simulink model "Trí"  (R2019a)
settings: Solver=FixedStepAuto  StartTime=0.0  StopTime=15  FixedStep=0.01  RelTol=1e-3
model workspace (MATLAB code in the model file):
  | Assem_DataFile.m
undefined symbols (not defined in the file): smiData, X, Y, Z
libraries: sm_lib x272, simulink x8, nesl_utility x8
(part 1 of 6)
settings Model: EnablePacing=on  Creator=DELL  LastModifiedBy=Minh Trí

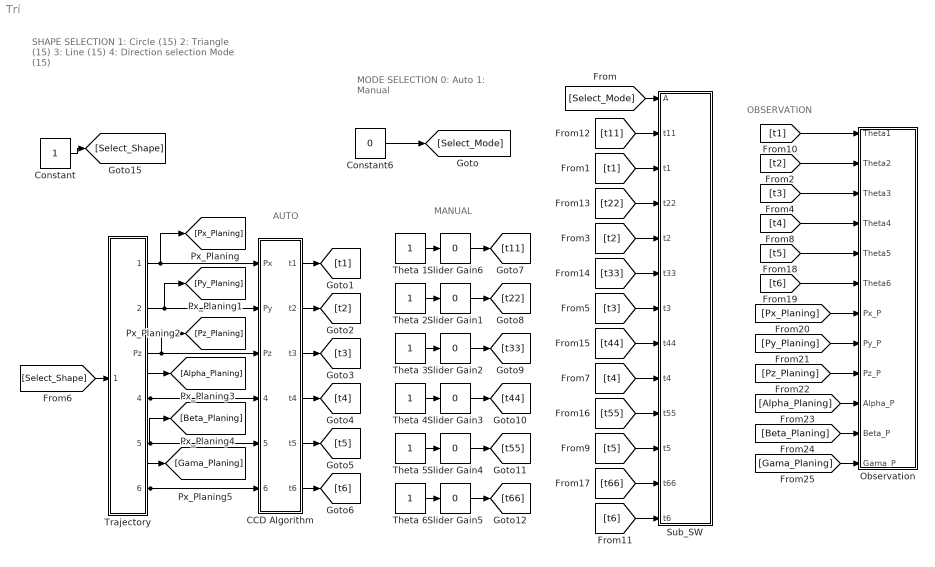
== system Trí ==
  note: MANUAL
  note: AUTO
  note: MODE SELECTION
      | 0: Auto
      | 1: Manual
  note: SHAPE SELECTION
      | 1: Circle (15)
      | 2: Triangle (15)
      | 3: Line (15)
      | 4: Direction selection Mode (15)
  note: OBSERVATION
  "CCD Algorithm " : MATLAB Function  TreatAsAtomicUnit=on
  Constant : Constant
  Constant6 : Constant  Value=0
  Observation : Subsystem
  Slider Gain1 : simulink/Math Operations/Slider Gain  gain=0  low=-30  high=45
  Slider Gain{2,4..6} (4 alike) : simulink/Math Operations/Slider Gain  gain=0  low=-45  high=45
  Slider Gain3 : simulink/Math Operations/Slider Gain  gain=0  low=-30  high=45
  Sub_SW : Subsystem
  "Theta 1 " : Constant
  "Theta 2 " : Constant
  Theta 3 : Constant
  "Theta 4 " : Constant
  "Theta 5 " : Constant
  Theta 6 : Constant
  "Trajectory " : Subsystem
  wires:
  Constant6/1 -> [Select_Mode]
  "Theta 1 "/1 -> Slider Gain6/1
  Slider Gain6/1 -> [t11]
  "Theta 2 "/1 -> Slider Gain1/1
  Slider Gain1/1 -> [t22]
  Theta 3/1 -> Slider Gain2/1
  Slider Gain2/1 -> [t33]
  "Theta 4 "/1 -> Slider Gain3/1
  "Theta 5 "/1 -> Slider Gain4/1
  Slider Gain3/1 -> [t44]
  Theta 6/1 -> Slider Gain5/1
  Slider Gain5/1 -> [t66]
  Slider Gain4/1 -> [t55]
  [t44] -> Sub_SW/8(t44)
  [t22] -> Sub_SW/4(t22)
  [t1] -> Sub_SW/3(t1)
  [t5] -> Sub_SW/11(t5)
  [Select_Mode] -> Sub_SW/1(A)
  [t3] -> Sub_SW/7(t3)
  [t4] -> Sub_SW/9(t4)
  [t66] -> Sub_SW/12(t66)
  [t2] -> Sub_SW/5(t2)
  [t33] -> Sub_SW/6(t33)
  [t6] -> Sub_SW/13(t6)
  [t55] -> Sub_SW/10(t55)
  [t11] -> Sub_SW/2(t11)
  "Trajectory "/1(Px) -> "CCD Algorithm "/1(Px), [Px_Planing]
  "CCD Algorithm "/6(t6) -> [t6]
  "CCD Algorithm "/5(t5) -> [t5]
  "CCD Algorithm "/4(t4) -> [t4]
  "CCD Algorithm "/3(t3) -> [t3]
  "CCD Algorithm "/2(t2) -> [t2]
  "CCD Algorithm "/1(t1) -> [t1]
  Constant/1 -> [Select_Shape]
  [Select_Shape] -> "Trajectory "/1(Shape)
  "Trajectory "/2(Py) -> "CCD Algorithm "/2(Py), [Py_Planing]
  "Trajectory "/3(Pz) -> "CCD Algorithm "/3(Pz), [Pz_Planing]
  "Trajectory "/4(Alpha) -> [Alpha_Planing], "CCD Algorithm "/4(alpha)
  "Trajectory "/5(Beta) -> [Beta_Planing], "CCD Algorithm "/5(beta)
  "Trajectory "/6(Gama) -> [Gama_Planing], "CCD Algorithm "/6(gama)
  [t1] -> Observation/1(Theta1)
  [t2] -> Observation/2(Theta2)
  [t3] -> Observation/3(Theta3)
  [t4] -> Observation/4(Theta4)
  [t5] -> Observation/5(Theta5)
  [t6] -> Observation/6(Theta6)
  [Alpha_Planing] -> Observation/10(Alpha_P)
  [Beta_Planing] -> Observation/11(Beta_P)
  [Pz_Planing] -> Observation/9(Pz_P)
  [Py_Planing] -> Observation/8(Py_P)
  [Px_Planing] -> Observation/7(Px_P)
  [Gama_Planing] -> Observation/12(Gama_P)

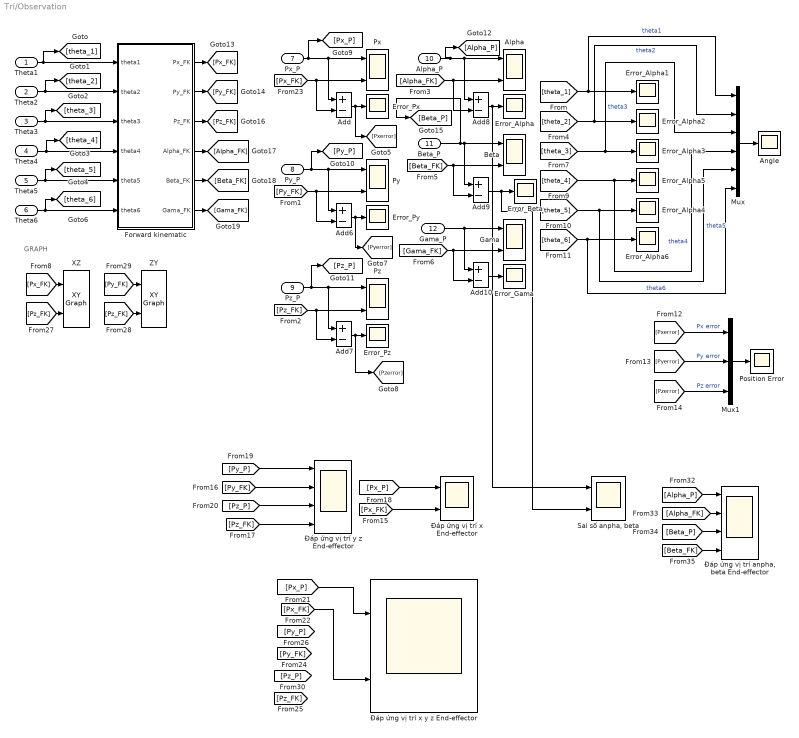
== system Trí/Observation ==
  note: GRAPH
  Theta1 : Inport
  Theta2 : Inport  Port=2
  Theta3 : Inport  Port=3
  Theta4 : Inport  Port=4
  Theta5 : Inport  Port=5
  Theta6 : Inport  Port=6
  Px_P : Inport  Port=7
  Py_P : Inport  Port=8
  Pz_P : Inport  Port=9
  Alpha_P : Inport  Port=10
  Beta_P : Inport  Port=11
  Gama_P : Inport  Port=12
  Add{,6..10} (6 alike) : Sum  Inputs=+-
  Alpha : Scope  NumInputPorts=2
  Angle : Scope
  Beta : Scope  NumInputPorts=2
  Error_Alpha{,1..6} (7 alike) : Scope
  Error_Beta : Scope
  Error_Gama : Scope
  Error_Px : Scope
  Error_Py : Scope
  Error_Pz : Scope
  "Forward kinematic " : MATLAB Function  TreatAsAtomicUnit=on
  Gama : Scope  NumInputPorts=2
  Mux : Mux  Inputs=6
  Mux1 : Mux  Inputs=3
  Position Error : Scope
  Px : Scope  NumInputPorts=2
  Py : Scope  NumInputPorts=2
  Pz : Scope  NumInputPorts=2
  "Sai số anpha, beta" : Scope  NumInputPorts=2
  XZ : simulink/Sinks/XY Graph  xmin=1000  xmax=1300  ymin=-150  ymax=150  st=0.01
  ZY : simulink/Sinks/XY Graph  xmin=-110  xmax=110  ymin=-90  ymax=90  st=0.01
  "Đáp ứng vị trí anpha, beta End-effector " : Scope  NumInputPorts=4
  Đáp ứng vị trí x End-effector : Scope  NumInputPorts=2
  Đáp ứng vị trí x y z End-effector : Scope  NumInputPorts=2
  "Đáp ứng vị trí y z End-effector " : Scope  NumInputPorts=4
  wires:
  [Py_FK] -> ZY/1
  [Px_FK] -> XZ/1
  [Pz_FK] -> XZ/2
  [Pz_FK] -> ZY/2
  Px_P/1 -> Add/1, Px/1, [Px_P]
  Add/1 -> [Pxerror], Error_Px/1
  [Px_FK] -> Px/2, Add/2
  "Forward kinematic "/4(Alpha_FK) -> [Alpha_FK]
  "Forward kinematic "/1(Px_FK) -> [Px_FK]
  "Forward kinematic "/2(Py_FK) -> [Py_FK]
  "Forward kinematic "/3(Pz_FK) -> [Pz_FK]
  "Forward kinematic "/6(Gama_FK) -> [Gama_FK]
  "Forward kinematic "/5(Beta_FK) -> [Beta_FK]
  Theta1/1 -> "Forward kinematic "/1(theta1), [theta_1]
  Theta2/1 -> [theta_2], "Forward kinematic "/2(theta2)
  Theta3/1 -> [theta_3], "Forward kinematic "/3(theta3)
  Theta4/1 -> [theta_4], "Forward kinematic "/4(theta4)
  Theta5/1 -> [theta_5], "Forward kinematic "/5(theta5)
  Theta6/1 -> [theta_6], "Forward kinematic "/6(theta6)
  [Py_FK] -> Add6/2, Py/2
  Add6/1 -> [Pyerror], Error_Py/1
  Py_P/1 -> [Py_P], Py/1, Add6/1
  Pz_P/1 -> [Pz_P], Add7/1, Pz/1
  Add7/1 -> [Pzerror], Error_Pz/1
  [Pz_FK] -> Add7/2, Pz/2
  [Alpha_FK] -> Add8/2, Alpha/2
  Add8/1 -> "Sai số anpha, beta"/1, Error_Alpha/1
  Alpha_P/1 -> [Alpha_P], Alpha/1, Add8/1
  Beta_P/1 -> [Beta_P], Add9/1, Beta/1
  [Beta_FK] -> Beta/2, Add9/2
  [Gama_FK] -> Add10/2, Gama/2
  Add10/1 -> Error_Gama/1
  Gama_P/1 -> Gama/1, Add10/1
  [theta_1] -> Mux/1, Error_Alpha1/1  "theta1"
  [theta_2] -> Mux/2, Error_Alpha2/1  "theta2"
  [theta_5] -> Mux/5, Error_Alpha4/1  "theta5"
  [theta_6] -> Mux/6, Error_Alpha6/1  "theta6"
  [theta_4] -> Mux/4, Error_Alpha5/1  "theta4"
  [theta_3] -> Mux/3, Error_Alpha3/1  "theta3"
  Mux/1 -> Angle/1
  Mux1/1 -> Position Error/1
  [Pxerror] -> Mux1/1  "Px error"
  [Pyerror] -> Mux1/2  "Py error"
  [Pzerror] -> Mux1/3  "Pz error"
  [Pz_P] -> "Đáp ứng vị trí y z End-effector "/3
  [Pz_FK] -> "Đáp ứng vị trí y z End-effector "/4
  [Px_P] -> Đáp ứng vị trí x End-effector/1
  [Px_FK] -> Đáp ứng vị trí x End-effector/2
  [Py_P] -> "Đáp ứng vị trí y z End-effector "/1
  [Py_FK] -> "Đáp ứng vị trí y z End-effector "/2
  Add9/1 -> "Sai số anpha, beta"/2, Error_Beta/1
  [Px_P] -> Đáp ứng vị trí x y z End-effector/1
  [Alpha_P] -> "Đáp ứng vị trí anpha, beta End-effector "/1
  [Alpha_FK] -> "Đáp ứng vị trí anpha, beta End-effector "/2
  [Beta_P] -> "Đáp ứng vị trí anpha, beta End-effector "/3
  [Beta_FK] -> "Đáp ứng vị trí anpha, beta End-effector "/4
  [Px_FK] -> Đáp ứng vị trí x y z End-effector/2

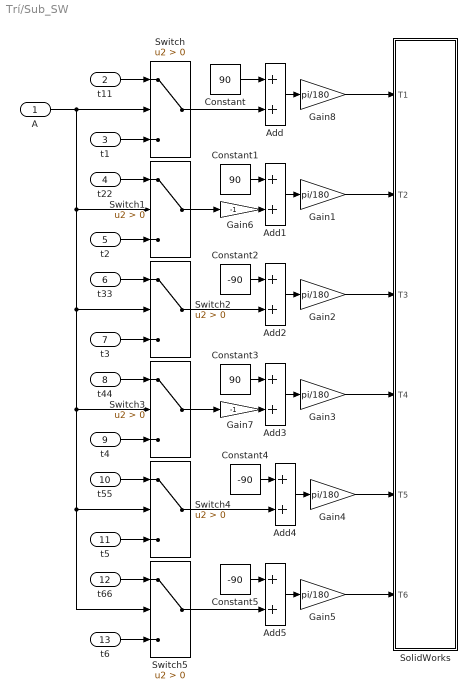
== system Trí/Sub_SW ==
  A : Inport
  t11 : Inport  Port=2
  t1 : Inport  Port=3
  t22 : Inport  Port=4
  t2 : Inport  Port=5
  t33 : Inport  Port=6
  t3 : Inport  Port=7
  t44 : Inport  Port=8
  t4 : Inport  Port=9
  t55 : Inport  Port=10
  t5 : Inport  Port=11
  t66 : Inport  Port=12
  t6 : Inport  Port=13
  Add{,1..5} (6 alike) : Sum
  Constant : Constant  Value=90
  Constant1 : Constant  Value=90
  Constant2 : Constant  Value=-90
  Constant3 : Constant  Value=90
  Constant4 : Constant  Value=-90
  Constant5 : Constant  Value=-90
  Gain{1..5,8} (6 alike) : Gain  Gain=pi/180
  Gain6 : Gain  Gain=-1
  Gain7 : Gain  Gain=-1
  SolidWorks : Subsystem
  Switch{,1..5} (6 alike) : Switch  Criteria=u2 > Threshold
  wires:
  Constant4/1 -> Add4/1
  Add4/1 -> Gain4/1
  Constant5/1 -> Add5/1
  Gain4/1 -> SolidWorks/5(T5)
  Add2/1 -> Gain2/1
  Switch3/1 -> Gain7/1
  Gain1/1 -> SolidWorks/2(T2)
  Add1/1 -> Gain1/1
  Constant/1 -> Add/1
  Gain8/1 -> SolidWorks/1(T1)
  Gain3/1 -> SolidWorks/4(T4)
  Gain7/1 -> Add3/2
  Add/1 -> Gain8/1
  Constant3/1 -> Add3/1
  Constant1/1 -> Add1/1
  Switch1/1 -> Gain6/1
  Switch/1 -> Add/2
  Gain5/1 -> SolidWorks/6(T6)
  Add5/1 -> Gain5/1
  Switch4/1 -> Add4/2
  Switch5/1 -> Add5/2
  Switch2/1 -> Add2/2
  Gain6/1 -> Add1/2
  Constant2/1 -> Add2/1
  Gain2/1 -> SolidWorks/3(T3)
  Add3/1 -> Gain3/1
  A/1 -> Switch5/2, Switch4/2, Switch3/2, Switch2/2, Switch1/2, Switch/2
  t11/1 -> Switch/1
  t22/1 -> Switch1/1
  t33/1 -> Switch2/1
  t44/1 -> Switch3/1
  t55/1 -> Switch4/1
  t66/1 -> Switch5/1
  t6/1 -> Switch5/3
  t5/1 -> Switch4/3
  t4/1 -> Switch3/3
  t3/1 -> Switch2/3
  t2/1 -> Switch1/3
  t1/1 -> Switch/3

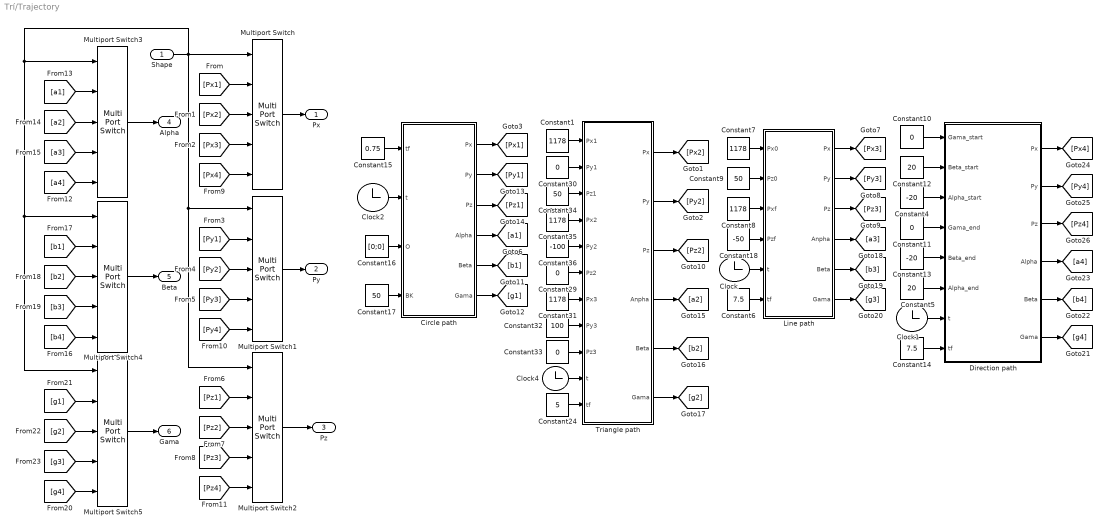
== system Trí/Trajectory  ==
  Shape : Inport
  Circle path : MATLAB Function  TreatAsAtomicUnit=on
  Clock{,1..2,4} (4 alike) : Clock
  Constant{1,7..8,31,35} (5 alike) : Constant  Value=1178
  Constant{10..11,29..30,33} (5 alike) : Constant  Value=0
  Constant12 : Constant  Value=20
  Constant13 : Constant  Value=-20
  Constant14 : Constant  Value=7.5
  Constant15 : Constant  Value=0.75
  Constant16 : Constant  Value=[0;0]
  Constant17 : Constant  Value=50
  Constant18 : Constant  Value=-50
  Constant24 : Constant  Value=5
  Constant32 : Constant  Value=100
  Constant34 : Constant  Value=50
  Constant36 : Constant  Value=-100
  Constant4 : Constant  Value=-20
  Constant5 : Constant  Value=20
  Constant6 : Constant  Value=7.5
  Constant9 : Constant  Value=50
  Direction path : MATLAB Function  TreatAsAtomicUnit=on
  Line path : MATLAB Function  TreatAsAtomicUnit=on
  Multiport Switch{,1..5} (6 alike) : MultiPortSwitch  Inputs=4
  Triangle path : MATLAB Function  TreatAsAtomicUnit=on
  Px : Outport
  Py : Outport  Port=2
  Pz : Outport  Port=3
  Alpha : Outport  Port=4
  Beta : Outport  Port=5
  Gama : Outport  Port=6
  wires:
  Multiport Switch1/1 -> Py/1
  Multiport Switch2/1 -> Pz/1
  Multiport Switch/1 -> Px/1
  Constant6/1 -> Line path/6(tf)
  Clock/1 -> Line path/5(t)
  Constant16/1 -> Circle path/3(O)
  Circle path/3(Pz) -> [Pz1]
  Constant15/1 -> Circle path/1(tf)
  Circle path/2(Py) -> [Py1]
  Constant9/1 -> Line path/2(Pz0)
  Line path/2(Py) -> [Py3]
  Clock2/1 -> Circle path/2(t)
  Circle path/1(Px) -> [Px1]
  Constant8/1 -> Line path/3(Pxf)
  Constant7/1 -> Line path/1(Px0)
  Line path/1(Px) -> [Px3]
  Constant18/1 -> Line path/4(Pzf)
  Constant17/1 -> Circle path/4(BK)
  Line path/3(Pz) -> [Pz3]
  [Px1] -> Multiport Switch/2
  [Px2] -> Multiport Switch/3
  [Px3] -> Multiport Switch/4
  [Py1] -> Multiport Switch1/2
  [Py2] -> Multiport Switch1/3
  [Py3] -> Multiport Switch1/4
  [Pz1] -> Multiport Switch2/2
  [Pz2] -> Multiport Switch2/3
  [Pz3] -> Multiport Switch2/4
  Triangle path/2(Py) -> [Py2]
  Triangle path/1(Px) -> [Px2]
  Constant36/1 -> Triangle path/5(Py2)
  Constant1/1 -> Triangle path/1(Px1)
  Constant24/1 -> Triangle path/11(tf)
  Constant29/1 -> Triangle path/6(Pz2)
  Constant32/1 -> Triangle path/8(Py3)
  Constant33/1 -> Triangle path/9(Pz3)
  Constant35/1 -> Triangle path/4(Px2)
  Constant34/1 -> Triangle path/3(Pz1)
  Clock4/1 -> Triangle path/10(t)
  Constant30/1 -> Triangle path/2(Py1)
  Constant31/1 -> Triangle path/7(Px3)
  [Px4] -> Multiport Switch/5
  [Py4] -> Multiport Switch1/5
  [Pz4] -> Multiport Switch2/5
  [a3] -> Multiport Switch3/4
  [a4] -> Multiport Switch3/5
  [a1] -> Multiport Switch3/2
  Multiport Switch3/1 -> Alpha/1
  [a2] -> Multiport Switch3/3
  [b3] -> Multiport Switch4/4
  [b4] -> Multiport Switch4/5
  [b1] -> Multiport Switch4/2
  Multiport Switch4/1 -> Beta/1
  [b2] -> Multiport Switch4/3
  Shape/1 -> Multiport Switch/1, Multiport Switch5/1, Multiport Switch4/1, Multiport Switch3/1, Multiport Switch2/1, Multiport Switch1/1
  [g3] -> Multiport Switch5/4
  [g4] -> Multiport Switch5/5
  [g1] -> Multiport Switch5/2
  Multiport Switch5/1 -> Gama/1
  [g2] -> Multiport Switch5/3
  Circle path/4(Alpha) -> [a1]
  Circle path/5(Beta) -> [b1]
  Circle path/6(Gama) -> [g1]
  Triangle path/3(Pz) -> [Pz2]
  Triangle path/4(Anpha) -> [a2]
  Triangle path/5(Beta) -> [b2]
  Triangle path/6(Gama) -> [g2]
  Line path/4(Anpha) -> [a3]
  Line path/5(Beta) -> [b3]
  Line path/6(Gama) -> [g3]
  Constant12/1 -> Direction path/2(Beta_start)
  Clock1/1 -> Direction path/7(t)
  Constant4/1 -> Direction path/3(Alpha_start)
  Direction path/4(Alpha) -> [a4]
  Direction path/5(Beta) -> [b4]
  Direction path/6(Gama) -> [g4]
  Constant5/1 -> Direction path/6(Alpha_end)
  Constant11/1 -> Direction path/4(Gama_end)
  Constant13/1 -> Direction path/5(Beta_end)
  Constant10/1 -> Direction path/1(Gama_start)
  Constant14/1 -> Direction path/8(tf)
  Direction path/1(Px) -> [Px4]
  Direction path/2(Py) -> [Py4]
  Direction path/3(Pz) -> [Pz4]

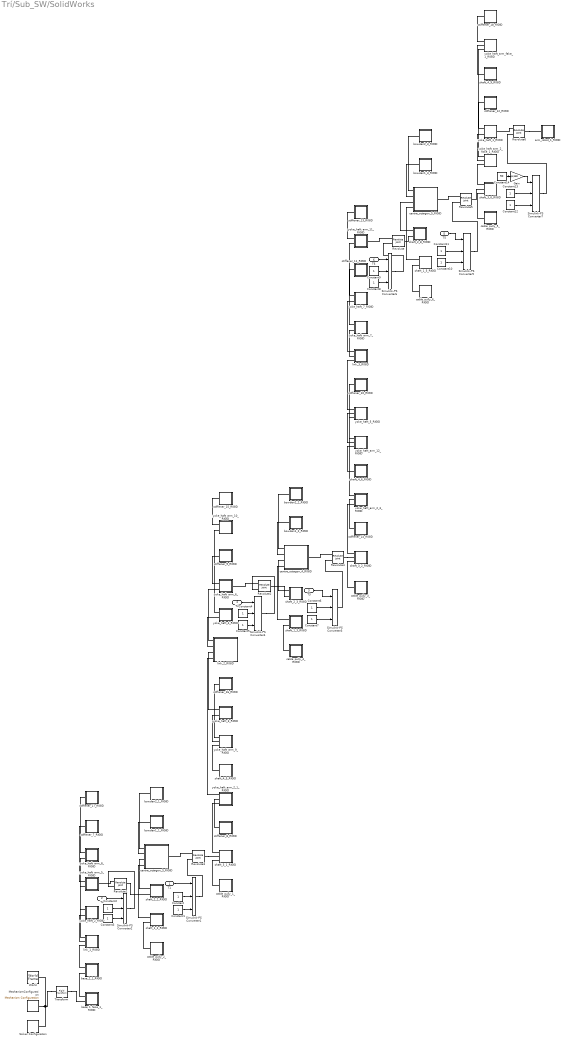
== system Trí/Sub_SW/SolidWorks ==
  T1 : Inport
  T2 : Inport  Port=2
  T3 : Inport  Port=3
  T4 : Inport  Port=4
  T5 : Inport  Port=5
  T6 : Inport  Port=6
  Constant{,1..13} (14 alike) : Constant
  Constant14 : Constant  Value=90
  Gain : Gain  Gain=pi/180
  MechanismConfiguration : sm_lib/Utilities/Mechanism Configuration  UniformGravity=Constant  GravityVector=[0 -9.80665 0]  GravityUnits=m/s^2  LinearizationDelta=0.001
  Revolute : sm_lib/Joints/Revolute Joint  SenseConstraintForce=off  SenseConstraintForceX=off  SenseConstraintForceY=off  SenseConstraintForceZ=off  SenseConstraintTorque=off  SenseConstraintTorqueX=off  SenseConstraintTorqueY=off  SenseConstraintTorqueZ=off  SenseTotalForce=off  SenseTotalForceX=off  SenseTotalForceY=off  SenseTotalForceZ=off  SenseTotalTorque=off  SenseTotalTorqueX=off  SenseTotalTorqueY=off  SenseTotalTorqueZ=off  CompositeWrenchDir=FollowerOnBase  CompositeWrenchFrame=BaseFrame  EquilibriumPosition=0  EquilibriumPositionUnits=rad  SpringStiffness=0  SpringStiffnessUnits=N*m/rad  DampingCoefficient=0  DampingCoefficientUnits=N*m/(rad/s)  TorqueActuationMode=ComputedTorque  MotionActuationMode=InputMotion  SensePosition=off  SenseVelocity=off  SenseAcceleration=off  SenseTorqueForce=off  SenseLowerLimitTorqueForce=off  SenseUpperLimitTorqueForce=off  LowerLimitSpecify=off  LowerLimitBound=-90  LowerLimitBoundUnits=deg  LowerLimitStiffness=1e4  LowerLimitStiffnessUnits=N*m/deg  LowerLimitDamping=10  LowerLimitDampingUnits=N*m/(deg/s)  LowerLimitTransitionRegionWidth=0.1  LowerLimitTransitionRegionWidthUnits=deg  UpperLimitSpecify=off  UpperLimitBound=90  UpperLimitBoundUnits=deg  UpperLimitStiffness=1e4  UpperLimitStiffnessUnits=N*m/deg  UpperLimitDamping=10  UpperLimitDampingUnits=N*m/(deg/s)  UpperLimitTransitionRegionWidth=0.1  UpperLimitTransitionRegionWidthUnits=deg  PositionTargetSpecify=on  PositionTargetPriority=Low  PositionTargetValue=smiData.RevoluteJoint(1).Rz.Pos  PositionTargetValueUnits=deg  VelocityTargetSpecify=off  VelocityTargetPriority=High  VelocityTargetValue=0  VelocityTargetValueUnits=deg/s
  Revolute1 : sm_lib/Joints/Revolute Joint  SenseConstraintForce=off  SenseConstraintForceX=off  SenseConstraintForceY=off  SenseConstraintForceZ=off  SenseConstraintTorque=off  SenseConstraintTorqueX=off  SenseConstraintTorqueY=off  SenseConstraintTorqueZ=off  SenseTotalForce=off  SenseTotalForceX=off  SenseTotalForceY=off  SenseTotalForceZ=off  SenseTotalTorque=off  SenseTotalTorqueX=off  SenseTotalTorqueY=off  SenseTotalTorqueZ=off  CompositeWrenchDir=FollowerOnBase  CompositeWrenchFrame=BaseFrame  EquilibriumPosition=0  EquilibriumPositionUnits=rad  SpringStiffness=0  SpringStiffnessUnits=N*m/rad  DampingCoefficient=0  DampingCoefficientUnits=N*m/(rad/s)  TorqueActuationMode=ComputedTorque  MotionActuationMode=InputMotion  SensePosition=off  SenseVelocity=off  SenseAcceleration=off  SenseTorqueForce=off  SenseLowerLimitTorqueForce=off  SenseUpperLimitTorqueForce=off  LowerLimitSpecify=off  LowerLimitBound=-90  LowerLimitBoundUnits=deg  LowerLimitStiffness=1e4  LowerLimitStiffnessUnits=N*m/deg  LowerLimitDamping=10  LowerLimitDampingUnits=N*m/(deg/s)  LowerLimitTransitionRegionWidth=0.1  LowerLimitTransitionRegionWidthUnits=deg  UpperLimitSpecify=off  UpperLimitBound=90  UpperLimitBoundUnits=deg  UpperLimitStiffness=1e4  UpperLimitStiffnessUnits=N*m/deg  UpperLimitDamping=10  UpperLimitDampingUnits=N*m/(deg/s)  UpperLimitTransitionRegionWidth=0.1  UpperLimitTransitionRegionWidthUnits=deg  PositionTargetSpecify=on  PositionTargetPriority=Low  PositionTargetValue=smiData.RevoluteJoint(2).Rz.Pos  PositionTargetValueUnits=deg  VelocityTargetSpecify=off  VelocityTargetPriority=High  VelocityTargetValue=0  VelocityTargetValueUnits=deg/s
  Revolute2 : sm_lib/Joints/Revolute Joint  SenseConstraintForce=off  SenseConstraintForceX=off  SenseConstraintForceY=off  SenseConstraintForceZ=off  SenseConstraintTorque=off  SenseConstraintTorqueX=off  SenseConstraintTorqueY=off  SenseConstraintTorqueZ=off  SenseTotalForce=off  SenseTotalForceX=off  SenseTotalForceY=off  SenseTotalForceZ=off  SenseTotalTorque=off  SenseTotalTorqueX=off  SenseTotalTorqueY=off  SenseTotalTorqueZ=off  CompositeWrenchDir=FollowerOnBase  CompositeWrenchFrame=BaseFrame  EquilibriumPosition=0  EquilibriumPositionUnits=rad  SpringStiffness=0  SpringStiffnessUnits=N*m/rad  DampingCoefficient=0  DampingCoefficientUnits=N*m/(rad/s)  TorqueActuationMode=ComputedTorque  MotionActuationMode=InputMotion  SensePosition=off  SenseVelocity=off  SenseAcceleration=off  SenseTorqueForce=off  SenseLowerLimitTorqueForce=off  SenseUpperLimitTorqueForce=off  LowerLimitSpecify=off  LowerLimitBound=-90  LowerLimitBoundUnits=deg  LowerLimitStiffness=1e4  LowerLimitStiffnessUnits=N*m/deg  LowerLimitDamping=10  LowerLimitDampingUnits=N*m/(deg/s)  LowerLimitTransitionRegionWidth=0.1  LowerLimitTransitionRegionWidthUnits=deg  UpperLimitSpecify=off  UpperLimitBound=90  UpperLimitBoundUnits=deg  UpperLimitStiffness=1e4  UpperLimitStiffnessUnits=N*m/deg  UpperLimitDamping=10  UpperLimitDampingUnits=N*m/(deg/s)  UpperLimitTransitionRegionWidth=0.1  UpperLimitTransitionRegionWidthUnits=deg  PositionTargetSpecify=on  PositionTargetPriority=Low  PositionTargetValue=smiData.RevoluteJoint(3).Rz.Pos  PositionTargetValueUnits=deg  VelocityTargetSpecify=off  VelocityTargetPriority=High  VelocityTargetValue=0  VelocityTargetValueUnits=deg/s
  Revolute3 : sm_lib/Joints/Revolute Joint  SenseConstraintForce=off  SenseConstraintForceX=off  SenseConstraintForceY=off  SenseConstraintForceZ=off  SenseConstraintTorque=off  SenseConstraintTorqueX=off  SenseConstraintTorqueY=off  SenseConstraintTorqueZ=off  SenseTotalForce=off  SenseTotalForceX=off  SenseTotalForceY=off  SenseTotalForceZ=off  SenseTotalTorque=off  SenseTotalTorqueX=off  SenseTotalTorqueY=off  SenseTotalTorqueZ=off  CompositeWrenchDir=FollowerOnBase  CompositeWrenchFrame=BaseFrame  EquilibriumPosition=0  EquilibriumPositionUnits=rad  SpringStiffness=0  SpringStiffnessUnits=N*m/rad  DampingCoefficient=0  DampingCoefficientUnits=N*m/(rad/s)  TorqueActuationMode=ComputedTorque  MotionActuationMode=InputMotion  SensePosition=off  SenseVelocity=off  SenseAcceleration=off  SenseTorqueForce=off  SenseLowerLimitTorqueForce=off  SenseUpperLimitTorqueForce=off  LowerLimitSpecify=off  LowerLimitBound=-90  LowerLimitBoundUnits=deg  LowerLimitStiffness=1e4  LowerLimitStiffnessUnits=N*m/deg  LowerLimitDamping=10  LowerLimitDampingUnits=N*m/(deg/s)  LowerLimitTransitionRegionWidth=0.1  LowerLimitTransitionRegionWidthUnits=deg  UpperLimitSpecify=off  UpperLimitBound=90  UpperLimitBoundUnits=deg  UpperLimitStiffness=1e4  UpperLimitStiffnessUnits=N*m/deg  UpperLimitDamping=10  UpperLimitDampingUnits=N*m/(deg/s)  UpperLimitTransitionRegionWidth=0.1  UpperLimitTransitionRegionWidthUnits=deg  PositionTargetSpecify=on  PositionTargetPriority=Low  PositionTargetValue=smiData.RevoluteJoint(4).Rz.Pos  PositionTargetValueUnits=deg  VelocityTargetSpecify=off  VelocityTargetPriority=High  VelocityTargetValue=0  VelocityTargetValueUnits=deg/s
  Revolute4 : sm_lib/Joints/Revolute Joint  SenseConstraintForce=off  SenseConstraintForceX=off  SenseConstraintForceY=off  SenseConstraintForceZ=off  SenseConstraintTorque=off  SenseConstraintTorqueX=off  SenseConstraintTorqueY=off  SenseConstraintTorqueZ=off  SenseTotalForce=off  SenseTotalForceX=off  SenseTotalForceY=off  SenseTotalForceZ=off  SenseTotalTorque=off  SenseTotalTorqueX=off  SenseTotalTorqueY=off  SenseTotalTorqueZ=off  CompositeWrenchDir=FollowerOnBase  CompositeWrenchFrame=BaseFrame  EquilibriumPosition=0  EquilibriumPositionUnits=rad  SpringStiffness=0  SpringStiffnessUnits=N*m/rad  DampingCoefficient=0  DampingCoefficientUnits=N*m/(rad/s)  TorqueActuationMode=ComputedTorque  MotionActuationMode=InputMotion  SensePosition=off  SenseVelocity=off  SenseAcceleration=off  SenseTorqueForce=off  SenseLowerLimitTorqueForce=off  SenseUpperLimitTorqueForce=off  LowerLimitSpecify=off  LowerLimitBound=-90  LowerLimitBoundUnits=deg  LowerLimitStiffness=1e4  LowerLimitStiffnessUnits=N*m/deg  LowerLimitDamping=10  LowerLimitDampingUnits=N*m/(deg/s)  LowerLimitTransitionRegionWidth=0.1  LowerLimitTransitionRegionWidthUnits=deg  UpperLimitSpecify=off  UpperLimitBound=90  UpperLimitBoundUnits=deg  UpperLimitStiffness=1e4  UpperLimitStiffnessUnits=N*m/deg  UpperLimitDamping=10  UpperLimitDampingUnits=N*m/(deg/s)  UpperLimitTransitionRegionWidth=0.1  UpperLimitTransitionRegionWidthUnits=deg  PositionTargetSpecify=on  PositionTargetPriority=Low  PositionTargetValue=smiData.RevoluteJoint(5).Rz.Pos  PositionTargetValueUnits=deg  VelocityTargetSpecify=off  VelocityTargetPriority=High  VelocityTargetValue=0  VelocityTargetValueUnits=deg/s
  Revolute5 : sm_lib/Joints/Revolute Joint  SenseConstraintForce=off  SenseConstraintForceX=off  SenseConstraintForceY=off  SenseConstraintForceZ=off  SenseConstraintTorque=off  SenseConstraintTorqueX=off  SenseConstraintTorqueY=off  SenseConstraintTorqueZ=off  SenseTotalForce=off  SenseTotalForceX=off  SenseTotalForceY=off  SenseTotalForceZ=off  SenseTotalTorque=off  SenseTotalTorqueX=off  SenseTotalTorqueY=off  SenseTotalTorqueZ=off  CompositeWrenchDir=FollowerOnBase  CompositeWrenchFrame=BaseFrame  EquilibriumPosition=0  EquilibriumPositionUnits=rad  SpringStiffness=0  SpringStiffnessUnits=N*m/rad  DampingCoefficient=0  DampingCoefficientUnits=N*m/(rad/s)  TorqueActuationMode=ComputedTorque  MotionActuationMode=InputMotion  SensePosition=off  SenseVelocity=off  SenseAcceleration=off  SenseTorqueForce=off  SenseLowerLimitTorqueForce=off  SenseUpperLimitTorqueForce=off  LowerLimitSpecify=off  LowerLimitBound=-90  LowerLimitBoundUnits=deg  LowerLimitStiffness=1e4  LowerLimitStiffnessUnits=N*m/deg  LowerLimitDamping=10  LowerLimitDampingUnits=N*m/(deg/s)  LowerLimitTransitionRegionWidth=0.1  LowerLimitTransitionRegionWidthUnits=deg  UpperLimitSpecify=off  UpperLimitBound=90  UpperLimitBoundUnits=deg  UpperLimitStiffness=1e4  UpperLimitStiffnessUnits=N*m/deg  UpperLimitDamping=10  UpperLimitDampingUnits=N*m/(deg/s)  UpperLimitTransitionRegionWidth=0.1  UpperLimitTransitionRegionWidthUnits=deg  PositionTargetSpecify=on  PositionTargetPriority=Low  PositionTargetValue=smiData.RevoluteJoint(6).Rz.Pos  PositionTargetValueUnits=deg  VelocityTargetSpecify=off  VelocityTargetPriority=High  VelocityTargetValue=0  VelocityTargetValueUnits=deg/s
  Revolute6 : sm_lib/Joints/Revolute Joint  SenseConstraintForce=off  SenseConstraintForceX=off  SenseConstraintForceY=off  SenseConstraintForceZ=off  SenseConstraintTorque=off  SenseConstraintTorqueX=off  SenseConstraintTorqueY=off  SenseConstraintTorqueZ=off  SenseTotalForce=off  SenseTotalForceX=off  SenseTotalForceY=off  SenseTotalForceZ=off  SenseTotalTorque=off  SenseTotalTorqueX=off  SenseTotalTorqueY=off  SenseTotalTorqueZ=off  CompositeWrenchDir=FollowerOnBase  CompositeWrenchFrame=BaseFrame  EquilibriumPosition=0  EquilibriumPositionUnits=rad  SpringStiffness=0  SpringStiffnessUnits=N*m/rad  DampingCoefficient=0  DampingCoefficientUnits=N*m/(rad/s)  TorqueActuationMode=ComputedTorque  MotionActuationMode=InputMotion  SensePosition=off  SenseVelocity=off  SenseAcceleration=off  SenseTorqueForce=off  SenseLowerLimitTorqueForce=off  SenseUpperLimitTorqueForce=off  LowerLimitSpecify=off  LowerLimitBound=-90  LowerLimitBoundUnits=deg  LowerLimitStiffness=1e4  LowerLimitStiffnessUnits=N*m/deg  LowerLimitDamping=10  LowerLimitDampingUnits=N*m/(deg/s)  LowerLimitTransitionRegionWidth=0.1  LowerLimitTransitionRegionWidthUnits=deg  UpperLimitSpecify=off  UpperLimitBound=90  UpperLimitBoundUnits=deg  UpperLimitStiffness=1e4  UpperLimitStiffnessUnits=N*m/deg  UpperLimitDamping=10  UpperLimitDampingUnits=N*m/(deg/s)  UpperLimitTransitionRegionWidth=0.1  UpperLimitTransitionRegionWidthUnits=deg  PositionTargetSpecify=on  PositionTargetPriority=Low  PositionTargetValue=smiData.RevoluteJoint(7).Rz.Pos  PositionTargetValueUnits=deg  VelocityTargetSpecify=off  VelocityTargetPriority=High  VelocityTargetValue=0  VelocityTargetValueUnits=deg/s
  Simulink-PS Converter1 : nesl_utility/Simulink-PS Converter  PhysicalDomain=network_engine_domain  SubClassName=ps_input  LeftPortType=input  RightPortType=output  PseudoPeriodic=off  Frequencies=[]  NoiseDistribution=none  NoiseParameters=[]  Unit=1  AffineConversion=on  FilteringAndDerivatives=provide  SimscapeFilterOrder=1  InputFilterTimeConstant=0.001  UdotUserProvided=2
  Simulink-PS Converter{2..7} (6 alike) : nesl_utility/Simulink-PS Converter  PhysicalDomain=network_engine_domain  SubClassName=ps_input  LeftPortType=input  RightPortType=output  PseudoPeriodic=off  Frequencies=[]  NoiseDistribution=none  NoiseParameters=[]  Unit=1  AffineConversion=off  FilteringAndDerivatives=provide  SimscapeFilterOrder=1  InputFilterTimeConstant=0.001  UdotUserProvided=2
  Solver Configuration : nesl_utility/Solver Configuration  PhysicalDomain=network_engine_domain  SubClassName=solver  LeftPortType=input  RightPortType=generic  Tones=[]  Harmonics=[]  SimulateNoise=off  Profile=off  UseLocalSampling=off  EnableSwitchedLinearOptims=on  FrequencyDomain=off  UseCCode=off  RelTol=0.001  AbsTol=1e-06  MinStep=1e-09  ToWorkspace=off  RevertToSquareIcSolve=off  NumHomotopyIterations=100  PhasorMode=off  PhasorModeNumHarmonics=1  DoDC=off  ResidualTolerance=1e-09  UseLocalSolver=off  LocalSolverChoice=NE_BACKWARD_EULER_ADVANCER  LocalSolverSampleTime=0.001  DoFixedCost=off  MaxNonlinIter=3  MaxModeIter=2  LinearAlgebra=auto  EquationFormulation=NE_TIME_EF  DelaysMemoryBudget=1024  AutomaticFiltering=on  FilteringTimeConstant=0.001  PartitionStorageMethod=AS_NEEDED  PartitionMemoryBudget=1024  PartitionMethod=ROBUST
  Transform : sm_lib/Frames and Transforms/Rigid Transform  TranslationMethod=Cartesian  TranslationStandardOffset=0  TranslationLengthUnit=mm  TranslationStandardAxis=+Z  TranslationCartesianOffset=smiData.RigidTransform(126).translation  TranslationROffset=0  TranslationROffsetUnits=m  TranslationZOffset=0  TranslationZOffsetUnits=m  TranslationThetaOffset=0  TranslationThetaOffsetUnits=deg  RotationMethod=ArbitraryAxis  RotationAngleUnits=rad  RotationStandardAxis=+Z  RotationAngle=smiData.RigidTransform(126).angle  RotationArbitraryAxis=smiData.RigidTransform(126).axis  FollAlignAxisA=+X  BaseAlignAxisA=+Y  FollAlignAxisB=+Y  BaseAlignAxisB=+Z  RotationSequenceAxes=FollowerAxes  RotationSequence=XYX  RotationSequenceAngles=[0 0 0]  RotationSequenceAnglesUnits=deg  RotationMatrix=[1 0 0; 0 1 0; 0 0 1]
  World : sm_lib/Frames and Transforms/World Frame
  arm_robot_1_RIGID : Subsystem
  base_1_fake_1_RIGID : Subsystem
  base_2_1_RIGID : Subsystem
  bowden1_1_RIGID : Subsystem
  bowden1_2_RIGID : Subsystem
  bowden1_3_RIGID : Subsystem
  bowden2_1_RIGID : Subsystem
  bowden2_2_RIGID : Subsystem
  bowden2_3_RIGID : Subsystem
  cable_pully_1_RIGID : Subsystem
  cable_pully_2_RIGID : Subsystem
  cable_pully_3_RIGID : Subsystem
  cable_pully_4_RIGID : Subsystem
  cable_pully_5_RIGID : Subsystem
  cable_pully_6_RIGID : Subsystem
  centre_octagon_3_RIGID : Subsystem
  centre_octagon_4_RIGID : Subsystem
  centre_octagon_5_RIGID : Subsystem
  link_1_RIGID : Subsystem
  link_2_RIGID : Subsystem
  link_3_RIGID : Subsystem
  shaft_1_2_RIGID : Subsystem
  shaft_1_3_RIGID : Subsystem
  shaft_1_5_RIGID : Subsystem
  shaft_2_2_RIGID : Subsystem
  shaft_2_3_RIGID : Subsystem
  shaft_2_8_RIGID : Subsystem
  shaft_3_1_RIGID : Subsystem
  shaft_3_2_RIGID : Subsystem
  shaft_3_6_RIGID : Subsystem
  shaft_4_5_RIGID : Subsystem
  shaft_4_6_RIGID : Subsystem
  shaft_4_9_RIGID : Subsystem
  stiffener_10_RIGID : Subsystem
  stiffener_11_RIGID : Subsystem
  stiffener_12_RIGID : Subsystem
  stiffener_13_RIGID : Subsystem
  stiffener_14_RIGID : Subsystem
  stiffener_15_RIGID : Subsystem
  stiffener_16_RIGID : Subsystem
  stiffener_17_RIGID : Subsystem
  stiffener_18_RIGID : Subsystem
  stiffener_7_RIGID : Subsystem
  stiffener_8_RIGID : Subsystem
  stiffener_9_RIGID : Subsystem
  yoke_haft_1_RIGID : Subsystem
  yoke_haft_2_RIGID : Subsystem
  yoke_haft_3_RIGID : Subsystem
  yoke_haft_4_RIGID : Subsystem
  yoke_haft_5_RIGID : Subsystem
  yoke_haft_7_RIGID : Subsystem
  yoke_haft_arm_10_RIGID : Subsystem
  yoke_haft_arm_11_RIGID : Subsystem
  yoke_haft_arm_12_RIGID : Subsystem
  yoke_haft_arm_2_1_RIGID : Subsystem
  yoke_haft_arm_2_3_RIGID : Subsystem
  yoke_haft_arm_2_fake_1_RIGID : Subsystem
  yoke_haft_arm_5_RIGID : Subsystem
  yoke_haft_arm_6_RIGID : Subsystem
  yoke_haft_arm_7_RIGID : Subsystem
  yoke_haft_arm_8_RIGID : Subsystem
  yoke_haft_arm_9_RIGID : Subsystem
  yoke_haft_arm_fake_1_RIGID : Subsystem
  wires:
  T1/1 -> Simulink-PS Converter1/1
  T2/1 -> Simulink-PS Converter2/1
  T3/1 -> Simulink-PS Converter3/1
  T6/1 -> Simulink-PS Converter6/1
  T4/1 -> Simulink-PS Converter4/1
  T5/1 -> Simulink-PS Converter5/1
  Constant1/1 -> Simulink-PS Converter1/3
  Constant/1 -> Simulink-PS Converter1/2
  Constant2/1 -> Simulink-PS Converter2/2
  Constant3/1 -> Simulink-PS Converter2/3
  Constant4/1 -> Simulink-PS Converter4/2
  Constant5/1 -> Simulink-PS Converter4/3
  Constant7/1 -> Simulink-PS Converter3/3
  Constant6/1 -> Simulink-PS Converter3/2
  Constant9/1 -> Simulink-PS Converter6/2
  Constant8/1 -> Simulink-PS Converter6/3
  Constant10/1 -> Simulink-PS Converter5/3
  Constant11/1 -> Simulink-PS Converter5/2
  Constant12/1 -> Simulink-PS Converter7/3
  Constant13/1 -> Simulink-PS Converter7/2
  Constant14/1 -> Gain/1
  Gain/1 -> Simulink-PS Converter7/1
  connections:
  Revolute3/RConn1 -- shaft_3_1_RIGID/LConn2
  yoke_haft_3_RIGID/LConn2 -- yoke_haft_arm_9_RIGID/LConn2
  Revolute5/LConn1 -- centre_octagon_5_RIGID/RConn1
  bowden2_1_RIGID/LConn1 -- centre_octagon_3_RIGID/LConn1
  stiffener_11_RIGID/LConn1 -- yoke_haft_arm_7_RIGID/LConn1
  yoke_haft_7_RIGID/LConn1 -- yoke_haft_arm_11_RIGID/LConn2
  centre_octagon_3_RIGID/LConn3 -- shaft_2_2_RIGID/LConn1
  Transform/LConn1 -- MechanismConfiguration/RConn1 -- Solver Configuration/RConn1 -- World/RConn1
  link_3_RIGID/LConn2 -- yoke_haft_arm_7_RIGID/LConn2
  stiffener_14_RIGID/LConn1 -- yoke_haft_arm_2_3_RIGID/LConn2
  Revolute5/RConn1 -- shaft_3_6_RIGID/LConn2
  stiffener_12_RIGID/LConn1 -- yoke_haft_arm_2_fake_1_RIGID/LConn1
  centre_octagon_5_RIGID/LConn3 -- shaft_2_8_RIGID/LConn1
  link_2_RIGID/LConn3 -- yoke_haft_3_RIGID/LConn1
  stiffener_10_RIGID/LConn1 -- yoke_haft_arm_12_RIGID/LConn1
  shaft_3_2_RIGID/LConn1 -- yoke_haft_arm_2_3_RIGID/LConn3
  shaft_3_1_RIGID/LConn1 -- yoke_haft_arm_2_1_RIGID/LConn3
  stiffener_7_RIGID/LConn1 -- yoke_haft_arm_5_RIGID/LConn1
  yoke_haft_1_RIGID/LConn1 -- yoke_haft_arm_fake_1_RIGID/LConn3
  shaft_4_6_RIGID/LConn1 -- yoke_haft_arm_12_RIGID/LConn3
  Revolute6/LConn1 -- yoke_haft_1_RIGID/RConn1
  link_1_RIGID/LConn1 -- yoke_haft_arm_5_RIGID/LConn2
  stiffener_8_RIGID/LConn1 -- yoke_haft_arm_2_1_RIGID/LConn2
  shaft_4_9_RIGID/LConn1 -- yoke_haft_arm_fake_1_RIGID/LConn2
  Revolute4/LConn1 -- centre_octagon_4_RIGID/RConn1
  Simulink-PS Converter5/RConn1 -- Revolute5/LConn2
  centre_octagon_4_RIGID/LConn4 -- shaft_1_3_RIGID/LConn1
  link_2_RIGID/LConn4 -- yoke_haft_arm_2_1_RIGID/LConn1
  cable_pully_3_RIGID/LConn1 -- shaft_3_2_RIGID/LConn3
  link_2_RIGID/LConn2 -- yoke_haft_4_RIGID/LConn2
  Revolute1/LConn1 -- yoke_haft_arm_5_RIGID/RConn1
  yoke_haft_4_RIGID/LConn1 -- yoke_haft_arm_10_RIGID/LConn2
  Revolute2/RConn1 -- shaft_2_3_RIGID/LConn2
  centre_octagon_3_RIGID/LConn4 -- shaft_1_2_RIGID/LConn1
  bowden2_3_RIGID/LConn1 -- centre_octagon_5_RIGID/LConn1
  yoke_haft_1_RIGID/LConn2 -- yoke_haft_arm_2_fake_1_RIGID/LConn2
  Revolute2/LConn1 -- yoke_haft_arm_6_RIGID/RConn1
  link_2_RIGID/LConn1 -- yoke_haft_arm_6_RIGID/LConn2
  cable_pully_6_RIGID/LConn1 -- shaft_1_5_RIGID/LConn2
  cable_pully_4_RIGID/LConn1 -- shaft_1_3_RIGID/LConn2
  link_3_RIGID/LConn1 -- yoke_haft_7_RIGID/LConn2
  Revolute4/RConn1 -- shaft_3_2_RIGID/LConn2
  Revolute3/LConn1 -- centre_octagon_3_RIGID/RConn1
  yoke_haft_5_RIGID/LConn2 -- yoke_haft_arm_12_RIGID/LConn2
  cable_pully_1_RIGID/LConn1 -- shaft_3_1_RIGID/LConn3
  Revolute6/RConn1 -- arm_robot_1_RIGID/LConn1
  Simulink-PS Converter1/RConn1 -- Revolute3/LConn2
  yoke_haft_5_RIGID/LConn3 -- yoke_haft_arm_2_3_RIGID/LConn1
  centre_octagon_4_RIGID/LConn3 -- shaft_2_3_RIGID/LConn1
  link_1_RIGID/LConn2 -- yoke_haft_2_RIGID/LConn2
  base_2_1_RIGID/LConn1 -- link_1_RIGID/LConn3
  stiffener_13_RIGID/LConn1 -- yoke_haft_arm_11_RIGID/LConn1
  cable_pully_5_RIGID/LConn1 -- shaft_3_6_RIGID/LConn3
  stiffener_9_RIGID/LConn1 -- yoke_haft_arm_6_RIGID/LConn1
  yoke_haft_2_RIGID/LConn1 -- yoke_haft_arm_8_RIGID/LConn2
  Simulink-PS Converter4/RConn1 -- Revolute2/LConn2
  shaft_4_5_RIGID/LConn1 -- yoke_haft_arm_9_RIGID/LConn3
  bowden1_1_RIGID/LConn1 -- centre_octagon_3_RIGID/LConn2
  link_3_RIGID/LConn3 -- yoke_haft_5_RIGID/LConn1
  shaft_3_6_RIGID/LConn1 -- yoke_haft_arm_2_fake_1_RIGID/LConn3
  stiffener_16_RIGID/LConn1 -- yoke_haft_arm_9_RIGID/LConn1
  bowden1_2_RIGID/LConn1 -- centre_octagon_4_RIGID/LConn2
  stiffener_18_RIGID/LConn1 -- yoke_haft_arm_fake_1_RIGID/LConn1
  centre_octagon_5_RIGID/LConn4 -- shaft_1_5_RIGID/LConn1
  base_1_fake_1_RIGID/LConn1 -- base_2_1_RIGID/LConn2
  stiffener_17_RIGID/LConn1 -- yoke_haft_arm_8_RIGID/LConn1
  bowden2_2_RIGID/LConn1 -- centre_octagon_4_RIGID/LConn1
  Revolute1/RConn1 -- shaft_2_2_RIGID/LConn2
  Revolute/LConn1 -- yoke_haft_arm_11_RIGID/RConn1
  Simulink-PS Converter6/RConn1 -- Revolute/LConn2
  Revolute/RConn1 -- shaft_2_8_RIGID/LConn2
  bowden1_3_RIGID/LConn1 -- centre_octagon_5_RIGID/LConn2
  stiffener_15_RIGID/LConn1 -- yoke_haft_arm_10_RIGID/LConn1
  Transform/RConn1 -- base_1_fake_1_RIGID/LConn2
  cable_pully_2_RIGID/LConn1 -- shaft_1_2_RIGID/LConn2
  Simulink-PS Converter3/RConn1 -- Revolute4/LConn2
  Simulink-PS Converter2/RConn1 -- Revolute1/LConn2
  Simulink-PS Converter7/RConn1 -- Revolute6/LConn2

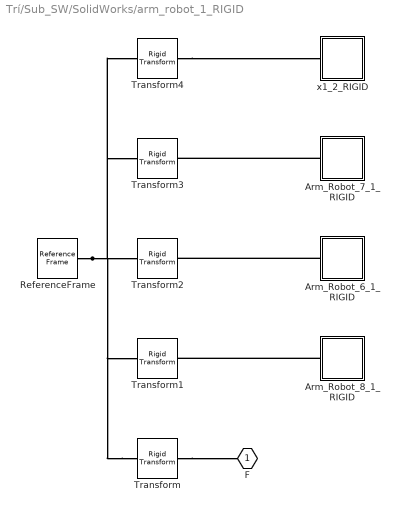
== system Trí/Sub_SW/SolidWorks/arm_robot_1_RIGID ==
  Arm_Robot_6_1_RIGID : Subsystem
  Arm_Robot_7_1_RIGID : Subsystem
  Arm_Robot_8_1_RIGID : Subsystem
  ReferenceFrame : sm_lib/Frames and Transforms/Reference Frame
  Transform : sm_lib/Frames and Transforms/Rigid Transform  TranslationMethod=Cartesian  TranslationStandardOffset=0  TranslationLengthUnit=mm  TranslationStandardAxis=+Z  TranslationCartesianOffset=smiData.RigidTransform(62).translation  TranslationROffset=0  TranslationROffsetUnits=m  TranslationZOffset=0  TranslationZOffsetUnits=m  TranslationThetaOffset=0  TranslationThetaOffsetUnits=deg  RotationMethod=ArbitraryAxis  RotationAngleUnits=rad  RotationStandardAxis=+Z  RotationAngle=smiData.RigidTransform(62).angle  RotationArbitraryAxis=smiData.RigidTransform(62).axis  FollAlignAxisA=+X  BaseAlignAxisA=+Y  FollAlignAxisB=+Y  BaseAlignAxisB=+Z  RotationSequenceAxes=FollowerAxes  RotationSequence=XYX  RotationSequenceAngles=[0 0 0]  RotationSequenceAnglesUnits=deg  RotationMatrix=[1 0 0; 0 1 0; 0 0 1]
  Transform1 : sm_lib/Frames and Transforms/Rigid Transform  TranslationMethod=Cartesian  TranslationStandardOffset=0  TranslationLengthUnit=mm  TranslationStandardAxis=+Z  TranslationCartesianOffset=smiData.RigidTransform(127).translation  TranslationROffset=0  TranslationROffsetUnits=m  TranslationZOffset=0  TranslationZOffsetUnits=m  TranslationThetaOffset=0  TranslationThetaOffsetUnits=deg  RotationMethod=ArbitraryAxis  RotationAngleUnits=rad  RotationStandardAxis=+Z  RotationAngle=smiData.RigidTransform(127).angle  RotationArbitraryAxis=smiData.RigidTransform(127).axis  FollAlignAxisA=+X  BaseAlignAxisA=+Y  FollAlignAxisB=+Y  BaseAlignAxisB=+Z  RotationSequenceAxes=FollowerAxes  RotationSequence=XYX  RotationSequenceAngles=[0 0 0]  RotationSequenceAnglesUnits=deg  RotationMatrix=[1 0 0; 0 1 0; 0 0 1]
  Transform2 : sm_lib/Frames and Transforms/Rigid Transform  TranslationMethod=Cartesian  TranslationStandardOffset=0  TranslationLengthUnit=mm  TranslationStandardAxis=+Z  TranslationCartesianOffset=smiData.RigidTransform(128).translation  TranslationROffset=0  TranslationROffsetUnits=m  TranslationZOffset=0  TranslationZOffsetUnits=m  TranslationThetaOffset=0  TranslationThetaOffsetUnits=deg  RotationMethod=ArbitraryAxis  RotationAngleUnits=rad  RotationStandardAxis=+Z  RotationAngle=smiData.RigidTransform(128).angle  RotationArbitraryAxis=smiData.RigidTransform(128).axis  FollAlignAxisA=+X  BaseAlignAxisA=+Y  FollAlignAxisB=+Y  BaseAlignAxisB=+Z  RotationSequenceAxes=FollowerAxes  RotationSequence=XYX  RotationSequenceAngles=[0 0 0]  RotationSequenceAnglesUnits=deg  RotationMatrix=[1 0 0; 0 1 0; 0 0 1]
  Transform3 : sm_lib/Frames and Transforms/Rigid Transform  TranslationMethod=Cartesian  TranslationStandardOffset=0  TranslationLengthUnit=mm  TranslationStandardAxis=+Z  TranslationCartesianOffset=smiData.RigidTransform(129).translation  TranslationROffset=0  TranslationROffsetUnits=m  TranslationZOffset=0  TranslationZOffsetUnits=m  TranslationThetaOffset=0  TranslationThetaOffsetUnits=deg  RotationMethod=ArbitraryAxis  RotationAngleUnits=rad  RotationStandardAxis=+Z  RotationAngle=smiData.RigidTransform(129).angle  RotationArbitraryAxis=smiData.RigidTransform(129).axis  FollAlignAxisA=+X  BaseAlignAxisA=+Y  FollAlignAxisB=+Y  BaseAlignAxisB=+Z  RotationSequenceAxes=FollowerAxes  RotationSequence=XYX  RotationSequenceAngles=[0 0 0]  RotationSequenceAnglesUnits=deg  RotationMatrix=[1 0 0; 0 1 0; 0 0 1]
  Transform4 : sm_lib/Frames and Transforms/Rigid Transform  TranslationMethod=Cartesian  TranslationStandardOffset=0  TranslationLengthUnit=mm  TranslationStandardAxis=+Z  TranslationCartesianOffset=smiData.RigidTransform(130).translation  TranslationROffset=0  TranslationROffsetUnits=m  TranslationZOffset=0  TranslationZOffsetUnits=m  TranslationThetaOffset=0  TranslationThetaOffsetUnits=deg  RotationMethod=ArbitraryAxis  RotationAngleUnits=rad  RotationStandardAxis=+Z  RotationAngle=smiData.RigidTransform(130).angle  RotationArbitraryAxis=smiData.RigidTransform(130).axis  FollAlignAxisA=+X  BaseAlignAxisA=+Y  FollAlignAxisB=+Y  BaseAlignAxisB=+Z  RotationSequenceAxes=FollowerAxes  RotationSequence=XYX  RotationSequenceAngles=[0 0 0]  RotationSequenceAnglesUnits=deg  RotationMatrix=[1 0 0; 0 1 0; 0 0 1]
  x1_2_RIGID : Subsystem
  F : PMIOPort  Side=Left
  connections:
  Transform/LConn1 -- ReferenceFrame/RConn1 -- Transform1/LConn1 -- Transform2/LConn1 -- Transform3/LConn1 -- Transform4/LConn1
  Transform/RConn1 -- F/RConn1
  Arm_Robot_8_1_RIGID/LConn1 -- Transform1/RConn1
  Arm_Robot_6_1_RIGID/LConn1 -- Transform2/RConn1
  Arm_Robot_7_1_RIGID/LConn1 -- Transform3/RConn1
  Transform4/RConn1 -- x1_2_RIGID/LConn1

== system Trí/Sub_SW/SolidWorks/base_1_fake_1_RIGID ==
  ReferenceFrame : sm_lib/Frames and Transforms/Reference Frame
  Solid : sm_lib/Body Elements/Solid  InertiaType=Custom  Mass=smiData.Solid(12).mass  MassUnits=kg  CenterOfMass=smiData.Solid(12).CoM  CenterOfMassUnits=mm  MomentsOfInertia=smiData.Solid(12).MoI  MomentsOfInertiaUnits=kg*mm^2  ProductsOfInertia=smiData.Solid(12).PoI  ProductsOfInertiaUnits=kg*mm^2  BasedOnType=Density  Density=1000  DensityUnits=kg/m^3  DoExposeReferenceFrame=on  SerializedFrames=<Frames/>  GraphicType=FromGeometry  MarkerShape=Sphere  MarkerSize=10  GraphicVisPropType=SimpleVisualProperties  GraphicDiffuseColor=smiData.Solid(12).color  GraphicSpecularColor=[0.5 0.5 0.5 1.0]  GraphicAmbientColor=[0.15 0.15 0.15 1.0]  GraphicEmissiveColor=[0.0 0.0 0.0 1.0]  GraphicShininess=75  GraphicOpacity=smiData.Solid(12).opacity  GeometryShape=FromFile  RectangleSize=[1 1]  RectangleSizeUnits=m  BrickDimensions=[1 1 1]  BrickDimensionUnits=m  CylinderRadius=1  CylinderRadiusUnits=m  CylinderLength=1  CylinderLengthUnits=m  SphereRadius=1  SphereRadiusUnits=m  EllipsoidRadii=[1 1 1]  EllipsoidRadiiUnits=m  ExtrusionCrossSection=[1 1; -1 1; -1 -1; 1 -1]  ExtrusionCrossSectionUnits=m  ExtrusionLength=1  ExtrusionLengthUnits=m  PolygonNumSides=3  PolygonOuterRadius=1  PolygonOuterRadiusUnits=m  ExtGeomFileType=STEP  ExtGeomFileName=base 1 fake_Default_sldprt.STEP  ExtGeomFileUnits=m  RevolutionCrossSection=[1 1; 1 -1; 2 -1; 2 1]  RevolutionCrossSectionUnits=m  RevolutionExtent=Full  RevolutionAngle=180  RevolutionAngleUnits=deg
  Transform : sm_lib/Frames and Transforms/Rigid Transform  TranslationMethod=Cartesian  TranslationStandardOffset=0  TranslationLengthUnit=mm  TranslationStandardAxis=+Z  TranslationCartesianOffset=smiData.RigidTransform(124).translation  TranslationROffset=0  TranslationROffsetUnits=m  TranslationZOffset=0  TranslationZOffsetUnits=m  TranslationThetaOffset=0  TranslationThetaOffsetUnits=deg  RotationMethod=ArbitraryAxis  RotationAngleUnits=rad  RotationStandardAxis=+Z  RotationAngle=smiData.RigidTransform(124).angle  RotationArbitraryAxis=smiData.RigidTransform(124).axis  FollAlignAxisA=+X  BaseAlignAxisA=+Y  FollAlignAxisB=+Y  BaseAlignAxisB=+Z  RotationSequenceAxes=FollowerAxes  RotationSequence=XYX  RotationSequenceAngles=[0 0 0]  RotationSequenceAnglesUnits=deg  RotationMatrix=[1 0 0; 0 1 0; 0 0 1]
  Transform1 : sm_lib/Frames and Transforms/Rigid Transform  TranslationMethod=Cartesian  TranslationStandardOffset=0  TranslationLengthUnit=mm  TranslationStandardAxis=+Z  TranslationCartesianOffset=smiData.RigidTransform(125).translation  TranslationROffset=0  TranslationROffsetUnits=m  TranslationZOffset=0  TranslationZOffsetUnits=m  TranslationThetaOffset=0  TranslationThetaOffsetUnits=deg  RotationMethod=ArbitraryAxis  RotationAngleUnits=rad  RotationStandardAxis=+Z  RotationAngle=smiData.RigidTransform(125).angle  RotationArbitraryAxis=smiData.RigidTransform(125).axis  FollAlignAxisA=+X  BaseAlignAxisA=+Y  FollAlignAxisB=+Y  BaseAlignAxisB=+Z  RotationSequenceAxes=FollowerAxes  RotationSequence=XYX  RotationSequenceAngles=[0 0 0]  RotationSequenceAnglesUnits=deg  RotationMatrix=[1 0 0; 0 1 0; 0 0 1]
  F : PMIOPort  Side=Left
  F1 : PMIOPort  Port=2  Side=Left
  connections:
  Solid/RConn1 -- ReferenceFrame/RConn1 -- Transform/LConn1 -- Transform1/LConn1
  Transform/RConn1 -- F/RConn1
  Transform1/RConn1 -- F1/RConn1

== system Trí/Sub_SW/SolidWorks/base_2_1_RIGID ==
  ReferenceFrame : sm_lib/Frames and Transforms/Reference Frame
  Solid : sm_lib/Body Elements/Solid  InertiaType=Custom  Mass=smiData.Solid(14).mass  MassUnits=kg  CenterOfMass=smiData.Solid(14).CoM  CenterOfMassUnits=mm  MomentsOfInertia=smiData.Solid(14).MoI  MomentsOfInertiaUnits=kg*mm^2  ProductsOfInertia=smiData.Solid(14).PoI  ProductsOfInertiaUnits=kg*mm^2  BasedOnType=Density  Density=1000  DensityUnits=kg/m^3  DoExposeReferenceFrame=on  SerializedFrames=<Frames/>  GraphicType=FromGeometry  MarkerShape=Sphere  MarkerSize=10  GraphicVisPropType=SimpleVisualProperties  GraphicDiffuseColor=smiData.Solid(14).color  GraphicSpecularColor=[0.5 0.5 0.5 1.0]  GraphicAmbientColor=[0.15 0.15 0.15 1.0]  GraphicEmissiveColor=[0.0 0.0 0.0 1.0]  GraphicShininess=75  GraphicOpacity=smiData.Solid(14).opacity  GeometryShape=FromFile  RectangleSize=[1 1]  RectangleSizeUnits=m  BrickDimensions=[1 1 1]  BrickDimensionUnits=m  CylinderRadius=1  CylinderRadiusUnits=m  CylinderLength=1  CylinderLengthUnits=m  SphereRadius=1  SphereRadiusUnits=m  EllipsoidRadii=[1 1 1]  EllipsoidRadiiUnits=m  ExtrusionCrossSection=[1 1; -1 1; -1 -1; 1 -1]  ExtrusionCrossSectionUnits=m  ExtrusionLength=1  ExtrusionLengthUnits=m  PolygonNumSides=3  PolygonOuterRadius=1  PolygonOuterRadiusUnits=m  ExtGeomFileType=STEP  ExtGeomFileName=base 2_Default_sldprt.STEP  ExtGeomFileUnits=m  RevolutionCrossSection=[1 1; 1 -1; 2 -1; 2 1]  RevolutionCrossSectionUnits=m  RevolutionExtent=Full  RevolutionAngle=180  RevolutionAngleUnits=deg
  Transform : sm_lib/Frames and Transforms/Rigid Transform  TranslationMethod=Cartesian  TranslationStandardOffset=0  TranslationLengthUnit=mm  TranslationStandardAxis=+Z  TranslationCartesianOffset=smiData.RigidTransform(77).translation  TranslationROffset=0  TranslationROffsetUnits=m  TranslationZOffset=0  TranslationZOffsetUnits=m  TranslationThetaOffset=0  TranslationThetaOffsetUnits=deg  RotationMethod=ArbitraryAxis  RotationAngleUnits=rad  RotationStandardAxis=+Z  RotationAngle=smiData.RigidTransform(77).angle  RotationArbitraryAxis=smiData.RigidTransform(77).axis  FollAlignAxisA=+X  BaseAlignAxisA=+Y  FollAlignAxisB=+Y  BaseAlignAxisB=+Z  RotationSequenceAxes=FollowerAxes  RotationSequence=XYX  RotationSequenceAngles=[0 0 0]  RotationSequenceAnglesUnits=deg  RotationMatrix=[1 0 0; 0 1 0; 0 0 1]
  Transform1 : sm_lib/Frames and Transforms/Rigid Transform  TranslationMethod=Cartesian  TranslationStandardOffset=0  TranslationLengthUnit=mm  TranslationStandardAxis=+Z  TranslationCartesianOffset=smiData.RigidTransform(123).translation  TranslationROffset=0  TranslationROffsetUnits=m  TranslationZOffset=0  TranslationZOffsetUnits=m  TranslationThetaOffset=0  TranslationThetaOffsetUnits=deg  RotationMethod=ArbitraryAxis  RotationAngleUnits=rad  RotationStandardAxis=+Z  RotationAngle=smiData.RigidTransform(123).angle  RotationArbitraryAxis=smiData.RigidTransform(123).axis  FollAlignAxisA=+X  BaseAlignAxisA=+Y  FollAlignAxisB=+Y  BaseAlignAxisB=+Z  RotationSequenceAxes=FollowerAxes  RotationSequence=XYX  RotationSequenceAngles=[0 0 0]  RotationSequenceAnglesUnits=deg  RotationMatrix=[1 0 0; 0 1 0; 0 0 1]
  F : PMIOPort  Side=Left
  F1 : PMIOPort  Port=2  Side=Left
  connections:
  Solid/RConn1 -- ReferenceFrame/RConn1 -- Transform/LConn1 -- Transform1/LConn1
  Transform/RConn1 -- F/RConn1
  Transform1/RConn1 -- F1/RConn1

== system Trí/Sub_SW/SolidWorks/bowden1_1_RIGID ==
  ReferenceFrame : sm_lib/Frames and Transforms/Reference Frame
  Solid : sm_lib/Body Elements/Solid  InertiaType=Custom  Mass=smiData.Solid(9).mass  MassUnits=kg  CenterOfMass=smiData.Solid(9).CoM  CenterOfMassUnits=mm  MomentsOfInertia=smiData.Solid(9).MoI  MomentsOfInertiaUnits=kg*mm^2  ProductsOfInertia=smiData.Solid(9).PoI  ProductsOfInertiaUnits=kg*mm^2  BasedOnType=Density  Density=1000  DensityUnits=kg/m^3  DoExposeReferenceFrame=on  SerializedFrames=<Frames/>  GraphicType=FromGeometry  MarkerShape=Sphere  MarkerSize=10  GraphicVisPropType=SimpleVisualProperties  GraphicDiffuseColor=smiData.Solid(9).color  GraphicSpecularColor=[0.5 0.5 0.5 1.0]  GraphicAmbientColor=[0.15 0.15 0.15 1.0]  GraphicEmissiveColor=[0.0 0.0 0.0 1.0]  GraphicShininess=75  GraphicOpacity=smiData.Solid(9).opacity  GeometryShape=FromFile  RectangleSize=[1 1]  RectangleSizeUnits=m  BrickDimensions=[1 1 1]  BrickDimensionUnits=m  CylinderRadius=1  CylinderRadiusUnits=m  CylinderLength=1  CylinderLengthUnits=m  SphereRadius=1  SphereRadiusUnits=m  EllipsoidRadii=[1 1 1]  EllipsoidRadiiUnits=m  ExtrusionCrossSection=[1 1; -1 1; -1 -1; 1 -1]  ExtrusionCrossSectionUnits=m  ExtrusionLength=1  ExtrusionLengthUnits=m  PolygonNumSides=3  PolygonOuterRadius=1  PolygonOuterRadiusUnits=m  ExtGeomFileType=STEP  ExtGeomFileName=bowden1_Default_sldprt.STEP  ExtGeomFileUnits=m  RevolutionCrossSection=[1 1; 1 -1; 2 -1; 2 1]  RevolutionCrossSectionUnits=m  RevolutionExtent=Full  RevolutionAngle=180  RevolutionAngleUnits=deg
  Transform : sm_lib/Frames and Transforms/Rigid Transform  TranslationMethod=Cartesian  TranslationStandardOffset=0  TranslationLengthUnit=mm  TranslationStandardAxis=+Z  TranslationCartesianOffset=smiData.RigidTransform(86).translation  TranslationROffset=0  TranslationROffsetUnits=m  TranslationZOffset=0  TranslationZOffsetUnits=m  TranslationThetaOffset=0  TranslationThetaOffsetUnits=deg  RotationMethod=ArbitraryAxis  RotationAngleUnits=rad  RotationStandardAxis=+Z  RotationAngle=smiData.RigidTransform(86).angle  RotationArbitraryAxis=smiData.RigidTransform(86).axis  FollAlignAxisA=+X  BaseAlignAxisA=+Y  FollAlignAxisB=+Y  BaseAlignAxisB=+Z  RotationSequenceAxes=FollowerAxes  RotationSequence=XYX  RotationSequenceAngles=[0 0 0]  RotationSequenceAnglesUnits=deg  RotationMatrix=[1 0 0; 0 1 0; 0 0 1]
  F : PMIOPort  Side=Left
  connections:
  Solid/RConn1 -- ReferenceFrame/RConn1 -- Transform/LConn1
  Transform/RConn1 -- F/RConn1
